simulink model "ssbdemo_frame"  (Simulink 8.3)
settings: Solver=FixedStepDiscrete  SolverMode=SingleTasking  StartTime=0.0  StopTime=99999999  RelTol=1e-3  AbsTol=1e-6
libraries: dspsrcs4 x2, dspxfrm3 x1, dspmisc x1, dspindex x1
settings Model: Creator=The MathWorks Inc.  CovMetricSettings=d  ExtModeTrigMode=oneshot  ExtModeArmWhenConnect=off
settings DataIOCC: LimitDataPoints=off  SaveOutput=off  SaveTime=off
settings OptimizationCC: BlockReduction=off  BooleanDataType=off  ExpressionDepthLimit=2147483647  RollThreshold=2  InitFltsAndDblsToZero=on
settings DebuggingCC: SaveWithParameterizedLinksMsg=none  SignalResolutionControl=TryResolveAllWithWarning  SolverPrmCheckMsg=none  MultiTaskDSMMsg=warning  MultiTaskCondExecSysMsg=none  IntegerOverflowMsg=none  FcnCallInpInsideContextMsg=UseLocalSettings  StrictBusMsg=None
settings HardwareCC: TargetUnknown=on
settings RTWCC: IncludeERTFirstTime=on
settings GRTTargetCC: TargetFcnLib=ansi_tfl_tmw.mat

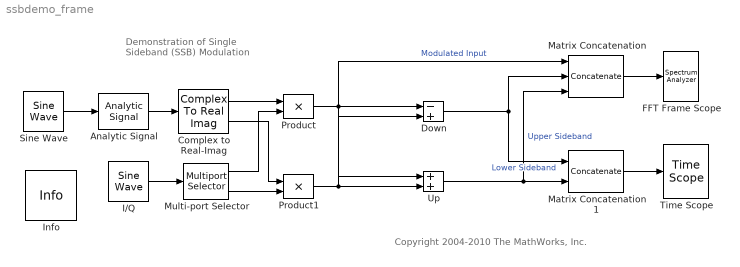
== system ssbdemo_frame ==
  note: Demonstration of
      | Single Sideband (SSB)
      | Modulation
  note: Copyright 2004-2010 The MathWorks, Inc.
  Analytic Signal : dspxfrm3/Analytic Signal  N=100  InputProcessing=Columns as channels (frame based)
  Complex to Real-Imag : ComplexToRealImag
  Down : Sum  Inputs=-+  SaturateOnIntegerOverflow=on  InputSameDT=on  OutDataTypeStr=Inherit: Same as first input
  FFT Frame Scope : SpectrumAnalyzer  ScopeSpecification=DataTag1
  I/Q : dspsrcs4/Sine Wave  Amplitude=1  Frequency=2  Phase=[0 pi/2]  SampleMode=Discrete  OutComplex=Real  CompMethod=Trigonometric fcn  TableSize=Speed  SampleTime=0.1  SamplesPerFrame=64  ResetState=Restart at time zero  dataType=double  wordLen=16  udDataType=sfix(16)  fracBitsMode=Best precision  numFracBits=15  OutDataTypeStr=double  LastOutDataTypeStr=double
  Info : dspmisc/Info  SystemSampleTime=-1
  Matrix Concatenation : Concatenate  NumInputs=3  Mode=Multidimensional array  ConcatenateDimension=2
  Matrix Concatenation1 : Concatenate  Mode=Multidimensional array  ConcatenateDimension=2
  Multi-port Selector : dspindex/Multiport Selector  rowsOrCols=Columns  idxCellArray={ 1, 2 }  idxErrMode=Clip Index
  Product : Product  SaturateOnIntegerOverflow=on  RndMeth=Zero  InputSameDT=on  OutDataTypeStr=Inherit: Same as first input
  Product1 : Product  SaturateOnIntegerOverflow=on  RndMeth=Zero  InputSameDT=on  OutDataTypeStr=Inherit: Same as first input
  Sine Wave : dspsrcs4/Sine Wave  Amplitude=1  Frequency=0.5  Phase=0  SampleMode=Discrete  OutComplex=Real  CompMethod=Trigonometric fcn  TableSize=Speed  SampleTime=0.1  SamplesPerFrame=64  ResetState=Restart at time zero  dataType=double  wordLen=16  udDataType=sfix(16)  fracBitsMode=Best precision  numFracBits=15  OutDataTypeStr=double  LastOutDataTypeStr=double
  Time Scope : TimeScope  DefaultConfigurationName=spbscopes.TimeScopeBlockCfg  ScopeSpecification=DataTag2
  Up : Sum  SaturateOnIntegerOverflow=on  InputSameDT=on  OutDataTypeStr=Inherit: Same as first input
  wires:
  Sine Wave/1 -> Analytic Signal/1
  Analytic Signal/1 -> Complex to Real-Imag/1
  Product/1 -> Down/1, Up/1, Matrix Concatenation/1  "Modulated Input"
  Product1/1 -> Up/2, Down/2
  Complex to Real-Imag/2 -> Product1/1
  Multi-port Selector/2 -> Product1/2
  Complex to Real-Imag/1 -> Product/1
  Multi-port Selector/1 -> Product/2
  Down/1 -> Matrix Concatenation1/1, Matrix Concatenation/2  "Lower Sideband"
  Up/1 -> Matrix Concatenation/3, Matrix Concatenation1/2  "Upper Sideband"
  I/Q/1 -> Multi-port Selector/1
  Matrix Concatenation/1 -> FFT Frame Scope/1
  Matrix Concatenation1/1 -> Time Scope/1
